simulink model "blackboxcl"  (R2014a)
settings: Solver=ode3  StartTime=0.0  StopTime=3  FixedStep=.001  RelTol=1e-3
values from neighbouring files (symbols this model uses):
  a = 21    [blackbox_step_graph.m]    (also in working.mat)
settings Model: Creator=gabriellemerritt  LastModifiedBy=gabriellemerritt

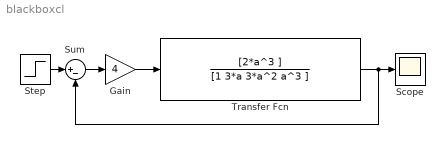
== system blackboxcl ==
  Gain : Gain  Gain=4
  Scope : Scope
      settings: TimeRange=3  YMin=0  YMax=1.8  SaveName=ScopeData2
  Step : Step  SampleTime=0
  Sum : Sum  Inputs=|+-
  Transfer Fcn : TransferFcn  Numerator=[2*a^3 ]  Denominator=[1 3*a 3*a^2 a^3 ]
  wires:
  Transfer Fcn/1 -> Scope/1, Sum/2
  Sum/1 -> Gain/1
  Gain/1 -> Transfer Fcn/1
  Step/1 -> Sum/1
